simulink model "rectifire_single_inverter_pv1"  (R2022b)
settings: Solver=ode23tb  StartTime=0  StopTime=3  RelTol=1e-4
undefined symbols (not defined in the file): Ion, Lithium, P_100, sigbuilder_block, time_step
libraries: spsSeriesRLCBranchLib x26, spsTriangleGeneratorLib x26, slpidlib x26, spsVoltageMeasurementLib x14, spsCurrentMeasurementLib x11, spsDiodeLib x9, simulink x8, spsIGBTDiodeLib x8, spsMosfetLib x8, powerlib_extras x4, spsGroundLib x2, spsBatteryLib x2
(part 1 of 6)
settings Model: Creator=Administrator  LastModifiedBy=Loki

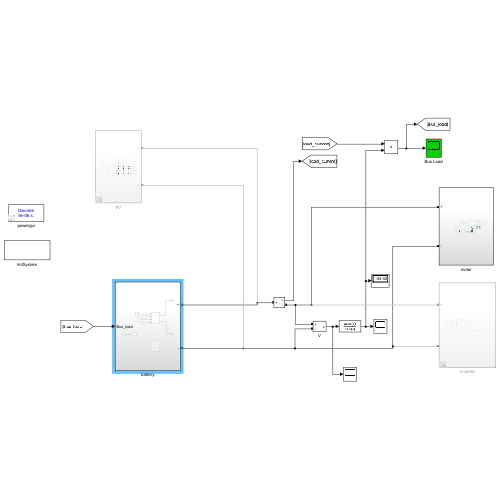
[thumbnail: Simulink's stored preview of the top-level diagram]
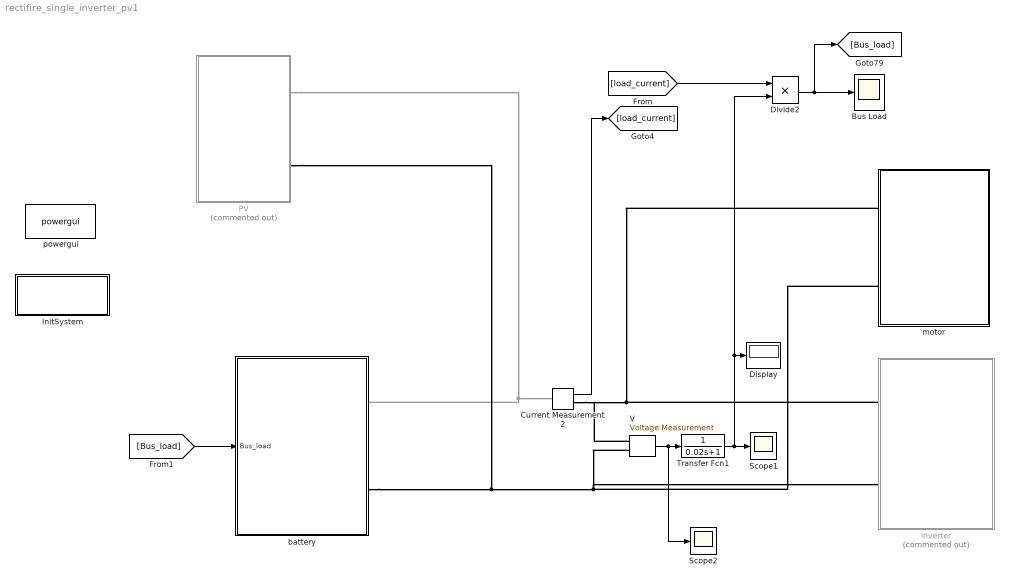
== system rectifire_single_inverter_pv1 ==
  Bus Load : Scope
  Current Measurement2 : spsCurrentMeasurementLib/Current Measurement  PhasorSimulation=off  OutputType=Complex  PSBequivalent=0
  Display : Display
  Divide2 : Product  Inputs=**
  InitSystem : Subsystem
      settings: OpenFcn=Battery_charge_discharge_FSBB_param_init
  PV : Subsystem  Commented=on
  Scope1 : Scope
  Scope2 : Scope
  Transfer Fcn1 : TransferFcn  Denominator=[0.02 1]
  V : spsVoltageMeasurementLib/Voltage Measurement  PhasorSimulation=off  OutputType=Complex  PSBequivalent=0
  battery : Subsystem
  inverter : Subsystem  Commented=on
  motor : Subsystem
  powergui : sps_lib/powergui  Priority=1  SimulationMode=Discrete  SampleTime=5e-6  frequency=60  Iterations=50  frequencyindice=0  Pbase=100e6  ErrMax=1e-4  UnitsV=kV  UnitsW=MW  buscounter=0  FunctionMessages=off  echomessages=off  EnableUseOfTLC=off  CurrentSourceSwitches=off  DisableSnubberDevices=off  DisableRonSwitches=off  DisableVfSwitches=off  DisplayEquations=off  AutomaticDiscreteSolvers=off  SolverType=Tustin/Backward Euler (TBE)  Interpol=off  ExternalGateDelay=off  methode=off  Ts=100  x0status=blocks  SPID=on  SwTol=0  HookPort=off  NonlinearTolerance=1e-4  nMaxIteration=100  ContinueOnMaxIteration=off  RestoreLinks=warning  ResistiveCurrentMeasurement=off  Frange=[0:2:500]  Ylog=off  Xlog=on  ShowGrid=off  save=off  variable=ZData  structure=0  ZoomFFT=off  StartTime=0.0  cycles=1  DisplayStyle=1  fundamental=60  FreqAxis=off  MaxFrequency=1000  frequencyindicesteady=1  RmsSteady=1  display=off
  wires:
  Transfer Fcn1/1 -> Divide2/2, Display/1, Scope1/1
  V/1 -> Scope2/1, Transfer Fcn1/1
  Current Measurement2/1 -> [load_current]
  [load_current] -> Divide2/1
  Divide2/1 -> Bus Load/1, [Bus_load]
  [Bus_load] -> battery/1(Bus_load)
  connections:
  PV/LConn1 -- battery/RConn1 -- Current Measurement2/LConn1
  battery/RConn2 -- motor/LConn2 -- inverter/LConn2 -- V/LConn2 -- PV/LConn2
  motor/LConn1 -- V/LConn1 -- Current Measurement2/RConn1 -- inverter/LConn1

== system rectifire_single_inverter_pv1/InitSystem ==

== system rectifire_single_inverter_pv1/PV ==
  C : spsSeriesRLCBranchLib/Series RLC Branch  LConnTagsString=__new0  RConnTagsString=__new0  BranchType=C  Resistance=0  Inductance=0  SetiL0=off  InitialCurrent=0  Capacitance=300e-6  Setx0=on  InitialVoltage=0  Measurements=None
  C1 : spsSeriesRLCBranchLib/Series RLC Branch  LConnTagsString=__new0  RConnTagsString=__new0  BranchType=C  Resistance=0  Inductance=0  SetiL0=off  InitialCurrent=0  Capacitance=300e-6  Setx0=off  InitialVoltage=0  Measurements=None
  Current Measurement : spsCurrentMeasurementLib/Current Measurement  PhasorSimulation=off  OutputType=Complex  PSBequivalent=0
  G : Subsystem  Tag=STV Subsys  LoadFcn=sigbuilder_block('load');  StartFcn=sigbuilder_block('start');  StopFcn=sigbuilder_block('stop');  ClipboardFcn=sigbuilder_block('clipboard');  mask(Sigbuilder block){tuvar=[0:10]}
      mask help: Sigbuilder GUI
      mask init:
      | if ~strcmp(get_param(bdroot(gcbh),'SimulationStatus'),'stopped') tuvar = sigbuilder_block('maskInit'); end
      settings: CopyFcn=sigbuilder_block('copy');  DeleteFcn=sigbuilder_block('delete');  ModelCloseFcn=sigbuilder_block('modelClose');  PreSaveFcn=sigbuilder_block('preSave');  PauseFcn=sigbuilder_block('pause')  ContinueFcn=sigbuilder_block('continue')  NameChangeFcn=sigbuilder_block('namechange');  OpenFcn=sigbuilder_block('open',[291 78 519 442.2 ]);  CloseFcn=sigbuilder_block('close');
      mask Display: plot(0, 0, 100, 100,[2, 2, 32, 32, 2], [68, 8, 8, 68, 68],[32, 2], [38, 38], [32, 19, 2],[53, 60, 44], [32, 17, 17, 2],[16, 16, 31, 31]);txt = getActiveGroup(gcbh);text(2, 100, txt,'verticalAlignment', 'top');
  Ground : spsGroundLib/Ground  LConnTagsString=a
  IGBT : spsIGBTLib/IGBT  Ron=0.00000001  Lon=0  Vf=1  Tf=1e-6  Tt=2e-6  IC=0  Rs=1e5  Cs=inf  Measurements=off
  L : spsSeriesRLCBranchLib/Series RLC Branch  LConnTagsString=__new0  RConnTagsString=__new0  BranchType=L  Resistance=0  Inductance=200e-6  SetiL0=off  InitialCurrent=1  Capacitance=inf  Setx0=off  InitialVoltage=0  Measurements=None
  "MPPT " : Subsystem
  PV module : Subsystem
  PWM : Subsystem
  R : spsSeriesRLCBranchLib/Series RLC Branch  Commented=on  LConnTagsString=__new0  RConnTagsString=__new0  BranchType=R  Resistance=30  Inductance=100e-6  SetiL0=off  InitialCurrent=0  Capacitance=inf  Setx0=off  InitialVoltage=0  Measurements=None
  Scope : Scope
  T : Subsystem  Tag=STV Subsys  LoadFcn=sigbuilder_block('load');  StartFcn=sigbuilder_block('start');  StopFcn=sigbuilder_block('stop');  ClipboardFcn=sigbuilder_block('clipboard');  mask(Sigbuilder block){tuvar=[0:10]}
      mask help: Sigbuilder GUI
      mask init:
      | if ~strcmp(get_param(bdroot(gcbh),'SimulationStatus'),'stopped') tuvar = sigbuilder_block('maskInit'); end
      settings: CopyFcn=sigbuilder_block('copy');  DeleteFcn=sigbuilder_block('delete');  ModelCloseFcn=sigbuilder_block('modelClose');  PreSaveFcn=sigbuilder_block('preSave');  PauseFcn=sigbuilder_block('pause')  ContinueFcn=sigbuilder_block('continue')  NameChangeFcn=sigbuilder_block('namechange');  OpenFcn=sigbuilder_block('open',[317 199.5 519.5 400 ]);  CloseFcn=sigbuilder_block('close');
      mask Display: plot(0, 0, 100, 100,[2, 2, 32, 32, 2], [68, 8, 8, 68, 68],[32, 2], [38, 38], [32, 19, 2],[53, 60, 44], [32, 17, 17, 2],[16, 16, 31, 31]);txt = getActiveGroup(gcbh);text(2, 100, txt,'verticalAlignment', 'top');
  Terminator{1..4} (4 alike) : Terminator
  VD : spsDiodeLib/Diode  Ron=0.00000001  Lon=0  Vf=0.7  IC=0  UseSnubber=off  Rs=500  Cs=250e-9  Measurements=off
  Voltage Measurement : spsVoltageMeasurementLib/Voltage Measurement  PhasorSimulation=off  OutputType=Complex  PSBequivalent=0
  Voltage Measurement1 : spsVoltageMeasurementLib/Voltage Measurement  PhasorSimulation=off  OutputType=Complex  PSBequivalent=0
  + : PMIOPort  Side=Left
  - : PMIOPort  Port=2  Side=Left
  wires:
  "MPPT "/4(D) -> Terminator1/1, PWM/1(D)  "D"
  Voltage Measurement1/1 -> Scope/1
  "MPPT "/3(I) -> Terminator4/1  "I"
  T/1(Signal 2) -> PV module/1(T)  "T"
  Current Measurement/1 -> "MPPT "/1(i)
  "MPPT "/2(U) -> Terminator3/1  "U"
  "MPPT "/1(P) -> Terminator2/1  "P"
  PWM/1(PWM) -> IGBT/1
  Voltage Measurement/1 -> PV module/3(Load Voltage), "MPPT "/2(u)
  G/1(Signal 1) -> PV module/2(G)  "G"
  connections:
  IGBT/RConn1 -- C/RConn1 -- -/RConn1 -- Voltage Measurement1/LConn2 -- R/RConn1 -- Voltage Measurement/LConn2 -- PV module/LConn1 -- Ground/LConn1 -- C1/RConn1
  R/LConn1 -- Voltage Measurement1/LConn1 -- +/RConn1 -- C/LConn1 -- VD/RConn1
  C1/LConn1 -- L/LConn1 -- Current Measurement/RConn1 -- Voltage Measurement/LConn1
  IGBT/LConn1 -- VD/LConn1 -- L/RConn1
  PV module/RConn1 -- Current Measurement/LConn1

== system rectifire_single_inverter_pv1/battery ==
  Bus_load : Inport
  Battery and DC-DC converter : Subsystem  Commented=on
  Battery and DC-DC converter1 : Subsystem
  Charge0 /Discharge1 : Step  Time=0.3  Before=1  SampleTime=0
  Constant19 : Constant  Value=96
  Constant2 : Constant  Value=30
  + : PMIOPort  Side=Right
  - : PMIOPort  Port=2  Side=Right
  wires:
  Bus_load/1 -> [Bus_load]
  [Bus_load] -> Battery and DC-DC converter1/4(Bus_load)
  Charge0 /Discharge1/1 -> Battery and DC-DC converter1/1(Mode=Charge0/DIscharge1)
  Constant2/1 -> Battery and DC-DC converter1/2(battery_I_charge_ref)
  Constant19/1 -> Battery and DC-DC converter1/3(V_bus_ref)
  connections:
  Battery and DC-DC converter1/RConn1 -- +/RConn1
  Battery and DC-DC converter1/RConn2 -- -/RConn1

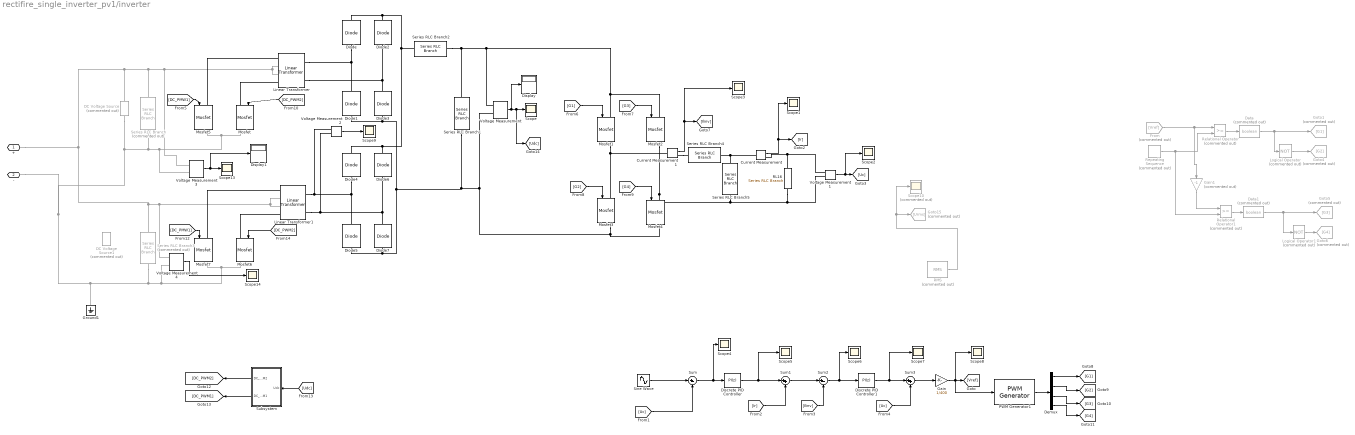
== system rectifire_single_inverter_pv1/inverter ==
  Current Measurement : spsCurrentMeasurementLib/Current Measurement  PhasorSimulation=off  OutputType=Complex  PSBequivalent=0
  Current Measurement1 : spsCurrentMeasurementLib/Current Measurement  PhasorSimulation=off  OutputType=Complex  PSBequivalent=0
  DC Voltage Source : spsDCVoltageSourceLib/DC Voltage Source  Commented=on  Amplitude=96  Measurements=None
  DC Voltage Source1 : spsDCVoltageSourceLib/DC Voltage Source  Commented=on  Amplitude=96  Measurements=None
  Data : DataTypeConversion  Commented=on  OutDataTypeStr=boolean  SaturateOnIntegerOverflow=off  RndMeth=Floor
  Data1 : DataTypeConversion  Commented=on  OutDataTypeStr=boolean  SaturateOnIntegerOverflow=off  RndMeth=Floor
  Demux : Demux
  Diode{,1..7} (8 alike) : spsDiodeLib/Diode  Ron=0.001  Lon=0  Vf=0.8  IC=0  UseSnubber=0  Rs=500  Cs=250e-9  Measurements=off
  Discrete PID Controller : slpidlib/PID Controller  Controller=PI  Form=Parallel  TimeDomain=Discrete-time  UseExternalTs=off  SampleTime=-1  IntegratorMethod=Forward Euler  FilterMethod=Forward Euler  ControllerParametersSource=internal  P=0.03115  I=21  UseKiTs=off  D=0  N=100  UseFilter=on  TunerSelectOption=Transfer Function Based (PID Tuner App)  InitialConditionSource=internal  InitialConditionForIntegrator=0  InitialConditionForFilter=0  DifferentiatorICPrevScaledInput=0  ExternalReset=none  TrackingMode=off  Kt=1  LimitOutput=off  SatLimitsSource=internal  UpperSaturationLimit=inf  LowerSaturationLimit=-inf  LinearizeAsGain=off  AntiWindupMode=none  Kb=1  LimitIntegrator=off  UpperIntegratorSaturationLimit=inf  LowerIntegratorSaturationLimit=-inf  POutMin=[]  POutMax=[]  IOutMin=[]  IOutMax=[]  DOutMin=[]  DOutMax=[]  NOutMin=[]  NOutMax=[]  SumOutMin=[]  SumOutMax=[]  SaturationOutMin=[]  SaturationOutMax=[]  PParamMin=[]  PParamMax=[]  IParamMin=[]  IParamMax=[]  DParamMin=[]  DParamMax=[]  NParamMin=[]  NParamMax=[]  KbParamMin=[]  KbParamMax=[]  KtParamMin=[]  KtParamMax=[]  KbOutMin=[]  KbOutMax=[]  KtOutMin=[]  KtOutMax=[]  IntegratorOutMin=[]  IntegratorOutMax=[]  FilterOutMin=[]  FilterOutMax=[]  SumI1OutMin=[]  SumI1OutMax=[]  SumI2OutMin=[]  SumI2OutMax=[]  SumI3OutMin=[]  SumI3OutMax=[]  SumI4OutMin=[]  SumI4OutMax=[]  SumDOutMin=[]  SumDOutMax=[]  DifferentiatorOutMin=[]  DifferentiatorOutMax=[]  FilterDiffOutCoefMin=[]  FilterDiffOutCoefMax=[]  ReciprocalOutMin=[]  ReciprocalOutMax=[]  SumDenOutMin=[]  SumDenOutMax=[]  SumNumOutMin=[]  SumNumOutMax=[]  DivideOutMin=[]  DivideOutMax=[]  UdiffTsProdOutMin=[]  UdiffTsProdOutMax=[]  NTsProdOutMin=[]  NTsProdOutMax=[]  UintegralTsProdOutMin=[]  UintegralTsProdOutMax=[]  UngainTsProdOutMin=[]  UngainTsProdOutMax=[]  ClampingZeroOutDataTypeStr=Inherit: Inherit via back propagation  ClampingZeroOutMin=[]  ClampingZeroOutMax=[]  FilterDenConstantOutDataTypeStr=Inherit: Inherit via back propagation  FilterDenConstantOutMin=[]  FilterDenConstantOutMax=[]  PCopyOutDataTypeStr=Inherit: Inherit via back propagation  PCopyOutMin=[]  PCopyOutMax=[]  NCopyOutDataTypeStr=Inherit: Inherit via back propagation  NCopyOutMin=[]  NCopyOutMax=[]  IntegratorContinuousStateAttributes=''  IntegratorStateMustResolveToSignalObject=off  IntegratorRTWStateStorageClass=Auto  FilterContinuousStateAttributes=''  FilterStateMustResolveToSignalObject=off  FilterRTWStateStorageClass=Auto  ParallelPVariant=InternalParameters  IdealPVariant=Disabled  IVariant=InternalParameters  DVariant=Disabled  IntegratorVariant=Discrete  SatVariant=Disabled  AWVariant=Passthrough  PCopyVariant=Disabled  TRVariant=Disabled  FdbkBlocksVariant=Forward  IdealPFdbkVariant=Disabled  SatFdbkVariant=Disabled  DerivativeFilterVariant=Disabled  NVariant=Disabled  NCopyVariant=Disabled_SignalSpec  FilterICVariant=Disabled  IntegratorICVariant=InternalICs  ExternalResetVariant=Disabled  TRSumVariant=Passthrough  SumFdbkVariant=Disabled  SumVariant=Sum_PI  TsampFilterVariant=InternalTs  TsampNgainVariant=Passthrough  TsampIntegralVariant=Passthrough  ExternalSaturationOutDataTypeStr=Inherit: Same as second input
      settings: LibrarySourceBlock=simulink/Discrete/Discrete PID Controller
  Discrete PID Controller1 : slpidlib/PID Controller  Controller=PI  Form=Parallel  TimeDomain=Discrete-time  UseExternalTs=off  SampleTime=-1  IntegratorMethod=Forward Euler  FilterMethod=Forward Euler  ControllerParametersSource=internal  P=27.066  I=6.67  UseKiTs=off  D=0  N=100  UseFilter=on  TunerSelectOption=Transfer Function Based (PID Tuner App)  InitialConditionSource=internal  InitialConditionForIntegrator=0  InitialConditionForFilter=0  DifferentiatorICPrevScaledInput=0  ExternalReset=none  TrackingMode=off  Kt=1  LimitOutput=off  SatLimitsSource=internal  UpperSaturationLimit=inf  LowerSaturationLimit=-inf  LinearizeAsGain=off  AntiWindupMode=none  Kb=1  LimitIntegrator=off  UpperIntegratorSaturationLimit=inf  LowerIntegratorSaturationLimit=-inf  POutMin=[]  POutMax=[]  IOutMin=[]  IOutMax=[]  DOutMin=[]  DOutMax=[]  NOutMin=[]  NOutMax=[]  SumOutMin=[]  SumOutMax=[]  SaturationOutMin=[]  SaturationOutMax=[]  PParamMin=[]  PParamMax=[]  IParamMin=[]  IParamMax=[]  DParamMin=[]  DParamMax=[]  NParamMin=[]  NParamMax=[]  KbParamMin=[]  KbParamMax=[]  KtParamMin=[]  KtParamMax=[]  KbOutMin=[]  KbOutMax=[]  KtOutMin=[]  KtOutMax=[]  IntegratorOutMin=[]  IntegratorOutMax=[]  FilterOutMin=[]  FilterOutMax=[]  SumI1OutMin=[]  SumI1OutMax=[]  SumI2OutMin=[]  SumI2OutMax=[]  SumI3OutMin=[]  SumI3OutMax=[]  SumI4OutMin=[]  SumI4OutMax=[]  SumDOutMin=[]  SumDOutMax=[]  DifferentiatorOutMin=[]  DifferentiatorOutMax=[]  FilterDiffOutCoefMin=[]  FilterDiffOutCoefMax=[]  ReciprocalOutMin=[]  ReciprocalOutMax=[]  SumDenOutMin=[]  SumDenOutMax=[]  SumNumOutMin=[]  SumNumOutMax=[]  DivideOutMin=[]  DivideOutMax=[]  UdiffTsProdOutMin=[]  UdiffTsProdOutMax=[]  NTsProdOutMin=[]  NTsProdOutMax=[]  UintegralTsProdOutMin=[]  UintegralTsProdOutMax=[]  UngainTsProdOutMin=[]  UngainTsProdOutMax=[]  ClampingZeroOutDataTypeStr=Inherit: Inherit via back propagation  ClampingZeroOutMin=[]  ClampingZeroOutMax=[]  FilterDenConstantOutDataTypeStr=Inherit: Inherit via back propagation  FilterDenConstantOutMin=[]  FilterDenConstantOutMax=[]  PCopyOutDataTypeStr=Inherit: Inherit via back propagation  PCopyOutMin=[]  PCopyOutMax=[]  NCopyOutDataTypeStr=Inherit: Inherit via back propagation  NCopyOutMin=[]  NCopyOutMax=[]  IntegratorContinuousStateAttributes=''  IntegratorStateMustResolveToSignalObject=off  IntegratorRTWStateStorageClass=Auto  FilterContinuousStateAttributes=''  FilterStateMustResolveToSignalObject=off  FilterRTWStateStorageClass=Auto  ParallelPVariant=InternalParameters  IdealPVariant=Disabled  IVariant=InternalParameters  DVariant=Disabled  IntegratorVariant=Discrete  SatVariant=Disabled  AWVariant=Passthrough  PCopyVariant=Disabled  TRVariant=Disabled  FdbkBlocksVariant=Forward  IdealPFdbkVariant=Disabled  SatFdbkVariant=Disabled  DerivativeFilterVariant=Disabled  NVariant=Disabled  NCopyVariant=Disabled_SignalSpec  FilterICVariant=Disabled  IntegratorICVariant=InternalICs  ExternalResetVariant=Disabled  TRSumVariant=Passthrough  SumFdbkVariant=Disabled  SumVariant=Sum_PI  TsampFilterVariant=InternalTs  TsampNgainVariant=Passthrough  TsampIntegralVariant=Passthrough  ExternalSaturationOutDataTypeStr=Inherit: Same as second input
      settings: LibrarySourceBlock=simulink/Discrete/Discrete PID Controller
  Display : Display
  Display1 : Display
  From : From  Commented=on  GotoTag=Vref
  Gain : Gain  Gain=1/400
  Gain1 : Gain  Commented=on  Gain=-1
  Goto1 : Goto  Commented=on  GotoTag=G1
  Goto15 : Goto  Commented=on  GotoTag=Urms
  Goto4 : Goto  Commented=on  GotoTag=G2
  Goto5 : Goto  Commented=on  GotoTag=G3
  Goto6 : Goto  Commented=on  GotoTag=G4
  Ground1 : spsGroundLib/Ground  LConnTagsString=a
  Linear Transformer : spsLinearTransformerLib/Linear Transformer  UNITS=SI  NominalPower=[ 3000 60 ]  winding1=[96 0 1e-6]  winding2=[96 0 1e-6]  ThreeWindings=on  winding3=[24 0 5e-6]  RmLm=[1.0804e+06 2866]  Measurements=None  DataType=on
  Linear Transformer1 : spsLinearTransformerLib/Linear Transformer  UNITS=SI  NominalPower=[ 3000 60 ]  winding1=[96 0 1e-6]  winding2=[96 0 1e-6]  ThreeWindings=on  winding3=[24 0 5e-6]  RmLm=[1.0804e+06 2866]  Measurements=None  DataType=on
  Logical Operator : Logic  Commented=on  Operator=NOT  AllPortsSameDT=off  OutDataTypeStr=boolean
  Logical Operator1 : Logic  Commented=on  Operator=NOT  AllPortsSameDT=off  OutDataTypeStr=boolean
  Mosfet{,1..7} (8 alike) : spsMosfetLib/Mosfet  Ron=0.1  Lon=0  Rd=0.01  Vfd=0  IC=0  Rs=1e5  Cs=inf  Measurements=on
  PWM Generator1 : powerlib_extras/Control  Blocks/PWM Generator  GeneratorMode="2-arm  bridge (4 pulses)"  Fc=10000  Internal=off  mIndex=0.4  Freq=60  Phase=0
      link override Triangle: rep_seq_y=[0 -1 1 0]
  RL16 : spsSeriesRLCBranchLib/Series RLC Branch  LConnTagsString=__new0  RConnTagsString=__new0  BranchType=R  Resistance=100  Inductance=1e-3  SetiL0=off  InitialCurrent=0  Capacitance=3000e-6  Setx0=off  InitialVoltage=0  Measurements=None
  RMS : spsRMSLib/RMS  Commented=on  TrueRMS=on  Freq=50  RMSInit=0  Ts=0
  Relational Operator : RelationalOperator  Commented=on  OutDataTypeStr=boolean  RndMeth=Simplest  InputSameDT=off
  Relational Operator1 : RelationalOperator  Commented=on  OutDataTypeStr=boolean  RndMeth=Simplest  InputSameDT=off
  Repeating Sequence : simulink/Sources/Repeating Sequence  Commented=on  rep_seq_t=[0 1/20000 1/10000]  rep_seq_y=[-1 1 -1]
  Scope{,1..9,13..14} (12 alike) : Scope
  Scope10 : Scope  Commented=on
  Series RLC Branch : spsSeriesRLCBranchLib/Series RLC Branch  Commented=on  LConnTagsString=__new0  RConnTagsString=__new0  BranchType=C  Resistance=1  Inductance=1e-3  SetiL0=off  InitialCurrent=0  Capacitance=1e-3  Setx0=off  InitialVoltage=0  Measurements=None
  Series RLC Branch1 : spsSeriesRLCBranchLib/Series RLC Branch  LConnTagsString=__new0  RConnTagsString=__new0  BranchType=C  Resistance=1  Inductance=1e-3  SetiL0=off  InitialCurrent=0  Capacitance=500e-6  Setx0=off  InitialVoltage=0  Measurements=None
  Series RLC Branch2 : spsSeriesRLCBranchLib/Series RLC Branch  LConnTagsString=__new0  RConnTagsString=__new0  BranchType=L  Resistance=1  Inductance=2e-3  SetiL0=off  InitialCurrent=0  Capacitance=1e-6  Setx0=off  InitialVoltage=0  Measurements=None
  Series RLC Branch3 : spsSeriesRLCBranchLib/Series RLC Branch  Commented=on  LConnTagsString=__new0  RConnTagsString=__new0  BranchType=C  Resistance=1  Inductance=1e-3  SetiL0=off  InitialCurrent=0  Capacitance=1e-3  Setx0=off  InitialVoltage=0  Measurements=None
  Series RLC Branch4 : spsSeriesRLCBranchLib/Series RLC Branch  LConnTagsString=__new0  RConnTagsString=__new0  BranchType=L  Resistance=0  Inductance=4.06e-3  SetiL0=off  InitialCurrent=0  Capacitance=1e-6  Setx0=off  InitialVoltage=0  Measurements=None
  Series RLC Branch5 : spsSeriesRLCBranchLib/Series RLC Branch  LConnTagsString=__new0  RConnTagsString=__new0  BranchType=C  Resistance=1  Inductance=1e-3  SetiL0=off  InitialCurrent=0  Capacitance=6.23e-6  Setx0=off  InitialVoltage=0  Measurements=None
  Sine Wave : Sin  Amplitude=311  Frequency=100*pi  SampleTime=0
  Subsystem : Subsystem
  Sum : Sum  Inputs=|+-
  Sum1 : Sum  Inputs=|++
  Sum2 : Sum  Inputs=|+-
  Sum3 : Sum  Inputs=|++
  Voltage Measurement{,1..4} (5 alike) : spsVoltageMeasurementLib/Voltage Measurement  PhasorSimulation=off  OutputType=Complex  PSBequivalent=0
  + : PMIOPort  Side=Left
  - : PMIOPort  Port=2  Side=Left
  wires:
  Current Measurement1/1 -> Scope3/1, [Ilinv]
  Logical Operator1/1 -> Goto6/1
  [G4] -> Mosfet4/1
  Repeating Sequence/1 -> Relational Operator1/2, Relational Operator/2
  Gain/1 -> PWM Generator1/1, Scope8/1, [Vref]
  [Ilinv] -> Sum2/2
  Voltage Measurement1/1 -> Scope2/1, [Uc]
  Sum1/1 -> Sum2/1
  [G3] -> Mosfet2/1
  Discrete PID Controller1/1 -> Scope7/1, Sum3/1
  RMS/1 -> Scope10/1, Goto15/1
  Voltage Measurement4/1 -> Scope14/1
  [DC_PWM2] -> Mosfet6/1
  Gain1/1 -> Relational Operator1/1
  Demux/3 -> [G3]
  [DC_PMW1] -> Mosfet7/1
  [G2] -> Mosfet3/1
  Sum/1 -> Scope4/1, Discrete PID Controller/1
  Relational Operator/1 -> Data/1
  Sine Wave/1 -> Sum/1
  Relational Operator1/1 -> Data1/1
  Data/1 -> Logical Operator/1, Goto1/1
  Sum3/1 -> Gain/1
  From/1 -> Gain1/1, Relational Operator/1
  Voltage Measurement3/1 -> Display1/1, Scope13/1
  Voltage Measurement/1 -> Display/1, [Udc], Scope/1
  [Uc] -> Sum3/2
  [Ir] -> Sum1/2
  [DC_PMW1] -> Mosfet5/1
  Current Measurement/1 -> Scope1/1, [Ir]
  Logical Operator/1 -> Goto4/1
  Sum2/1 -> Scope6/1, Discrete PID Controller1/1
  PWM Generator1/1 -> Demux/1
  [G1] -> Mosfet1/1
  Discrete PID Controller/1 -> Scope5/1, Sum1/1
  Demux/1 -> [G1]
  Demux/4 -> [G4]
  [DC_PWM2] -> Mosfet/1
  Voltage Measurement2/1 -> Scope9/1
  Data1/1 -> Logical Operator1/1, Goto5/1
  Demux/2 -> [G2]
  [Uc] -> Sum/2
  [Udc] -> Subsystem/1(Udc)
  Subsystem/1(DC_PWM2) -> [DC_PWM2]
  Subsystem/2(DC_PWM1) -> [DC_PWM1]
  connections:
  RL16/RConn1 -- Voltage Measurement1/LConn2 -- Series RLC Branch5/RConn1 -- Mosfet2/RConn1 -- Mosfet4/LConn1
  Linear Transformer/LConn1 -- Diode1/RConn1 -- Diode/LConn1
  Diode4/LConn1 -- Diode5/RConn1 -- Voltage Measurement2/LConn1 -- Linear Transformer1/LConn1
  Current Measurement/LConn1 -- Series RLC Branch5/LConn1 -- Series RLC Branch4/LConn1
  Voltage Measurement/LConn2 -- Mosfet3/RConn1 -- Mosfet4/RConn1 -- Series RLC Branch1/RConn1 -- Diode5/LConn1 -- Diode7/LConn1 -- Diode1/LConn1 -- Diode3/LConn1
  Mosfet1/RConn1 -- Current Measurement1/LConn1 -- Mosfet3/LConn1
  Diode7/RConn1 -- Diode6/LConn1 -- Voltage Measurement2/LConn2 -- Linear Transformer1/LConn2
  Voltage Measurement/LConn1 -- Series RLC Branch2/LConn1 -- Series RLC Branch1/LConn1 -- Mosfet1/LConn1 -- Mosfet2/LConn1
  Series RLC Branch/LConn1 -- Voltage Measurement3/LConn1 -- Linear Transformer/RConn3 -- Linear Transformer/RConn2 -- DC Voltage Source/RConn1 -- Series RLC Branch3/LConn1 -- Voltage Measurement4/LConn1 -- Linear Transformer1/RConn2 -- Linear Transformer1/RConn3 -- +/RConn1
  Diode6/RConn1 -- Series RLC Branch2/RConn1 -- Diode/RConn1 -- Diode2/RConn1 -- Diode4/RConn1
  Linear Transformer/LConn2 -- Diode2/LConn1 -- Diode3/RConn1
  RL16/LConn1 -- Voltage Measurement1/LConn1 -- Current Measurement/RConn1
  DC Voltage Source/LConn1 -- -/RConn1 -- Ground1/LConn1 -- Series RLC Branch3/RConn1 -- Voltage Measurement4/LConn2 -- Mosfet7/RConn1 -- Mosfet6/RConn1 -- Mosfet5/RConn1 -- Mosfet/RConn1 -- Voltage Measurement3/LConn2 -- Series RLC Branch/RConn1
  Current Measurement1/RConn1 -- Series RLC Branch4/RConn1
  Linear Transformer1/RConn1 -- Mosfet7/LConn1
  Mosfet5/LConn1 -- Linear Transformer/RConn1
  Mosfet/LConn1 -- Linear Transformer/RConn4
  Linear Transformer1/RConn4 -- Mosfet6/LConn1

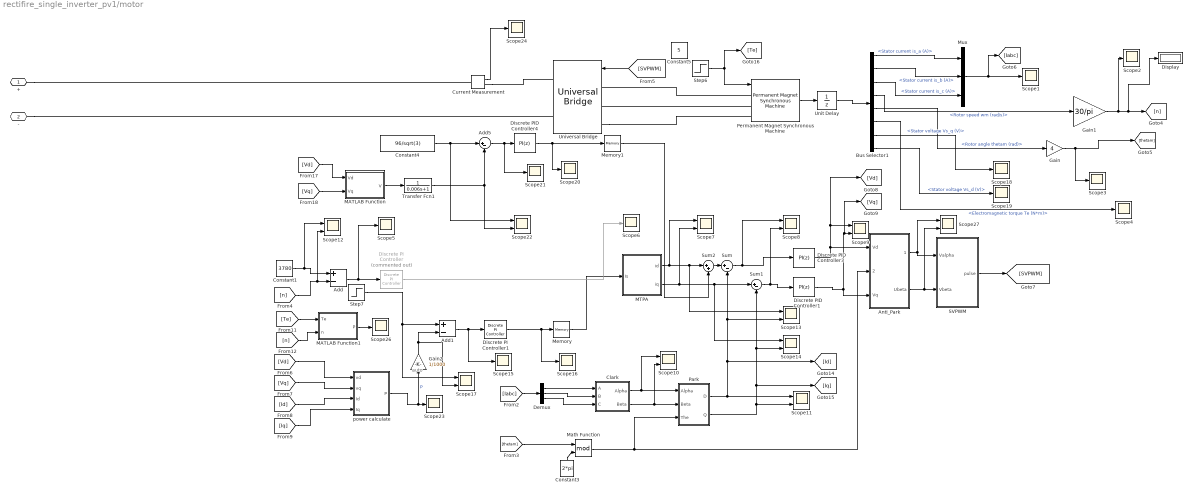
== system rectifire_single_inverter_pv1/motor ==
  note: auto
  Add : Sum  Inputs=+-
  Add1 : Sum  Inputs=+-
  Add5 : Sum  Inputs=|+-
  Anti_Park : Subsystem
  Bus Selector1 : BusSelector  OutputSignals=Stator current is_a (A),Stator current is_b (A),Stator current is_c (A),Rotor speed wm (rad/s),Rotor angle thetam (rad),Electromagnetic torque Te (N*m),Stator voltage Vs_q (V),Stator voltage Vs_d (V)
  Clark : Subsystem
  Constant1 : Constant  Value=3780
  Constant3 : Constant  Value=2*pi  SampleTime=5e-6
  Constant4 : Constant  Value=96/sqrt(3)
  Constant5 : Constant  Value=5
  Current Measurement : spsCurrentMeasurementLib/Current Measurement  PhasorSimulation=off  OutputType=Complex  PSBequivalent=0
  Demux : Demux  Outputs=3
  Discrete PI Controller : powerlib_extras/Discrete  Control Blocks/Discrete PI Controller  Commented=on  Kp=1.7  Ki=0.2  Par_Limits=[100 -100]  Init=0  Ts=5e-6
  Discrete PI Controller1 : powerlib_extras/Discrete  Control Blocks/Discrete PI Controller  Kp=20  Ki=500  Par_Limits=[inf -inf]  Init=0  Ts=5e-6
  Discrete PID Controller1 : slpidlib/PID Controller  Controller=PI  Form=Parallel  TimeDomain=Discrete-time  UseExternalTs=off  SampleTime=5e-6  IntegratorMethod=Forward Euler  FilterMethod=Forward Euler  ControllerParametersSource=internal  P=1.2  I=0.1  UseKiTs=off  D=0  N=100  UseFilter=on  TunerSelectOption=Transfer Function Based (PID Tuner App)  InitialConditionSource=internal  InitialConditionForIntegrator=0  InitialConditionForFilter=0  DifferentiatorICPrevScaledInput=0  ExternalReset=none  TrackingMode=off  Kt=1  LimitOutput=on  SatLimitsSource=internal  UpperSaturationLimit=50  LowerSaturationLimit=-50  LinearizeAsGain=off  AntiWindupMode=none  Kb=1  LimitIntegrator=off  UpperIntegratorSaturationLimit=inf  LowerIntegratorSaturationLimit=-inf  POutMin=[]  POutMax=[]  IOutMin=[]  IOutMax=[]  DOutMin=[]  DOutMax=[]  NOutMin=[]  NOutMax=[]  SumOutMin=[]  SumOutMax=[]  SaturationOutMin=[]  SaturationOutMax=[]  PParamMin=[]  PParamMax=[]  IParamMin=[]  IParamMax=[]  DParamMin=[]  DParamMax=[]  NParamMin=[]  NParamMax=[]  KbParamMin=[]  KbParamMax=[]  KtParamMin=[]  KtParamMax=[]  KbOutMin=[]  KbOutMax=[]  KtOutMin=[]  KtOutMax=[]  IntegratorOutMin=[]  IntegratorOutMax=[]  FilterOutMin=[]  FilterOutMax=[]  SumI1OutMin=[]  SumI1OutMax=[]  SumI2OutMin=[]  SumI2OutMax=[]  SumI3OutMin=[]  SumI3OutMax=[]  SumI4OutMin=[]  SumI4OutMax=[]  SumDOutMin=[]  SumDOutMax=[]  DifferentiatorOutMin=[]  DifferentiatorOutMax=[]  FilterDiffOutCoefMin=[]  FilterDiffOutCoefMax=[]  ReciprocalOutMin=[]  ReciprocalOutMax=[]  SumDenOutMin=[]  SumDenOutMax=[]  SumNumOutMin=[]  SumNumOutMax=[]  DivideOutMin=[]  DivideOutMax=[]  UdiffTsProdOutMin=[]  UdiffTsProdOutMax=[]  NTsProdOutMin=[]  NTsProdOutMax=[]  UintegralTsProdOutMin=[]  UintegralTsProdOutMax=[]  UngainTsProdOutMin=[]  UngainTsProdOutMax=[]  ClampingZeroOutDataTypeStr=Inherit: Inherit via back propagation  ClampingZeroOutMin=[]  ClampingZeroOutMax=[]  FilterDenConstantOutDataTypeStr=Inherit: Inherit via back propagation  FilterDenConstantOutMin=[]  FilterDenConstantOutMax=[]  PCopyOutDataTypeStr=Inherit: Inherit via back propagation  PCopyOutMin=[]  PCopyOutMax=[]  NCopyOutDataTypeStr=Inherit: Inherit via back propagation  NCopyOutMin=[]  NCopyOutMax=[]  IntegratorContinuousStateAttributes=''  IntegratorStateMustResolveToSignalObject=off  IntegratorRTWStateStorageClass=Auto  FilterContinuousStateAttributes=''  FilterStateMustResolveToSignalObject=off  FilterRTWStateStorageClass=Auto  ParallelPVariant=InternalParameters  IdealPVariant=Disabled  IVariant=InternalParameters  DVariant=Disabled  IntegratorVariant=Discrete  SatVariant=Enabled  AWVariant=Passthrough  PCopyVariant=Disabled  TRVariant=Disabled  FdbkBlocksVariant=Forward  IdealPFdbkVariant=Disabled  SatFdbkVariant=Disabled  DerivativeFilterVariant=Disabled  NVariant=Disabled  NCopyVariant=Disabled_SignalSpec  FilterICVariant=Disabled  IntegratorICVariant=InternalICs  ExternalResetVariant=Disabled  TRSumVariant=Passthrough  SumFdbkVariant=Disabled  SumVariant=Sum_PI  TsampFilterVariant=InternalTs  TsampNgainVariant=Passthrough  TsampIntegralVariant=Passthrough  ExternalSaturationOutDataTypeStr=Inherit: Same as second input
  Discrete PID Controller3 : slpidlib/PID Controller  Controller=PI  Form=Parallel  TimeDomain=Discrete-time  UseExternalTs=off  SampleTime=5e-6  IntegratorMethod=Forward Euler  FilterMethod=Forward Euler  ControllerParametersSource=internal  P=1.2  I=0.1  UseKiTs=off  D=0  N=100  UseFilter=on  TunerSelectOption=Transfer Function Based (PID Tuner App)  InitialConditionSource=internal  InitialConditionForIntegrator=0  InitialConditionForFilter=0  DifferentiatorICPrevScaledInput=0  ExternalReset=none  TrackingMode=off  Kt=1  LimitOutput=on  SatLimitsSource=internal  UpperSaturationLimit=50  LowerSaturationLimit=-50  LinearizeAsGain=off  AntiWindupMode=none  Kb=1  LimitIntegrator=off  UpperIntegratorSaturationLimit=inf  LowerIntegratorSaturationLimit=-inf  POutMin=[]  POutMax=[]  IOutMin=[]  IOutMax=[]  DOutMin=[]  DOutMax=[]  NOutMin=[]  NOutMax=[]  SumOutMin=[]  SumOutMax=[]  SaturationOutMin=[]  SaturationOutMax=[]  PParamMin=[]  PParamMax=[]  IParamMin=[]  IParamMax=[]  DParamMin=[]  DParamMax=[]  NParamMin=[]  NParamMax=[]  KbParamMin=[]  KbParamMax=[]  KtParamMin=[]  KtParamMax=[]  KbOutMin=[]  KbOutMax=[]  KtOutMin=[]  KtOutMax=[]  IntegratorOutMin=[]  IntegratorOutMax=[]  FilterOutMin=[]  FilterOutMax=[]  SumI1OutMin=[]  SumI1OutMax=[]  SumI2OutMin=[]  SumI2OutMax=[]  SumI3OutMin=[]  SumI3OutMax=[]  SumI4OutMin=[]  SumI4OutMax=[]  SumDOutMin=[]  SumDOutMax=[]  DifferentiatorOutMin=[]  DifferentiatorOutMax=[]  FilterDiffOutCoefMin=[]  FilterDiffOutCoefMax=[]  ReciprocalOutMin=[]  ReciprocalOutMax=[]  SumDenOutMin=[]  SumDenOutMax=[]  SumNumOutMin=[]  SumNumOutMax=[]  DivideOutMin=[]  DivideOutMax=[]  UdiffTsProdOutMin=[]  UdiffTsProdOutMax=[]  NTsProdOutMin=[]  NTsProdOutMax=[]  UintegralTsProdOutMin=[]  UintegralTsProdOutMax=[]  UngainTsProdOutMin=[]  UngainTsProdOutMax=[]  ClampingZeroOutDataTypeStr=Inherit: Inherit via back propagation  ClampingZeroOutMin=[]  ClampingZeroOutMax=[]  FilterDenConstantOutDataTypeStr=Inherit: Inherit via back propagation  FilterDenConstantOutMin=[]  FilterDenConstantOutMax=[]  PCopyOutDataTypeStr=Inherit: Inherit via back propagation  PCopyOutMin=[]  PCopyOutMax=[]  NCopyOutDataTypeStr=Inherit: Inherit via back propagation  NCopyOutMin=[]  NCopyOutMax=[]  IntegratorContinuousStateAttributes=''  IntegratorStateMustResolveToSignalObject=off  IntegratorRTWStateStorageClass=Auto  FilterContinuousStateAttributes=''  FilterStateMustResolveToSignalObject=off  FilterRTWStateStorageClass=Auto  ParallelPVariant=InternalParameters  IdealPVariant=Disabled  IVariant=InternalParameters  DVariant=Disabled  IntegratorVariant=Discrete  SatVariant=Enabled  AWVariant=Passthrough  PCopyVariant=Disabled  TRVariant=Disabled  FdbkBlocksVariant=Forward  IdealPFdbkVariant=Disabled  SatFdbkVariant=Disabled  DerivativeFilterVariant=Disabled  NVariant=Disabled  NCopyVariant=Disabled_SignalSpec  FilterICVariant=Disabled  IntegratorICVariant=InternalICs  ExternalResetVariant=Disabled  TRSumVariant=Passthrough  SumFdbkVariant=Disabled  SumVariant=Sum_PI  TsampFilterVariant=InternalTs  TsampNgainVariant=Passthrough  TsampIntegralVariant=Passthrough  ExternalSaturationOutDataTypeStr=Inherit: Same as second input
  Discrete PID Controller4 : slpidlib/PID Controller  Controller=PI  Form=Parallel  TimeDomain=Discrete-time  UseExternalTs=off  SampleTime=5e-6  IntegratorMethod=Forward Euler  FilterMethod=Forward Euler  ControllerParametersSource=internal  P=0.02  I=0.000008  UseKiTs=off  D=0  N=100  UseFilter=on  TunerSelectOption=Transfer Function Based (PID Tuner App)  InitialConditionSource=internal  InitialConditionForIntegrator=0  InitialConditionForFilter=0  DifferentiatorICPrevScaledInput=0  ExternalReset=none  TrackingMode=off  Kt=1  LimitOutput=off  SatLimitsSource=internal  UpperSaturationLimit=inf  LowerSaturationLimit=-inf  LinearizeAsGain=off  AntiWindupMode=none  Kb=1  LimitIntegrator=off  UpperIntegratorSaturationLimit=inf  LowerIntegratorSaturationLimit=-inf  POutMin=[]  POutMax=[]  IOutMin=[]  IOutMax=[]  DOutMin=[]  DOutMax=[]  NOutMin=[]  NOutMax=[]  SumOutMin=[]  SumOutMax=[]  SaturationOutMin=[]  SaturationOutMax=[]  PParamMin=[]  PParamMax=[]  IParamMin=[]  IParamMax=[]  DParamMin=[]  DParamMax=[]  NParamMin=[]  NParamMax=[]  KbParamMin=[]  KbParamMax=[]  KtParamMin=[]  KtParamMax=[]  KbOutMin=[]  KbOutMax=[]  KtOutMin=[]  KtOutMax=[]  IntegratorOutMin=[]  IntegratorOutMax=[]  FilterOutMin=[]  FilterOutMax=[]  SumI1OutMin=[]  SumI1OutMax=[]  SumI2OutMin=[]  SumI2OutMax=[]  SumI3OutMin=[]  SumI3OutMax=[]  SumI4OutMin=[]  SumI4OutMax=[]  SumDOutMin=[]  SumDOutMax=[]  DifferentiatorOutMin=[]  DifferentiatorOutMax=[]  FilterDiffOutCoefMin=[]  FilterDiffOutCoefMax=[]  ReciprocalOutMin=[]  ReciprocalOutMax=[]  SumDenOutMin=[]  SumDenOutMax=[]  SumNumOutMin=[]  SumNumOutMax=[]  DivideOutMin=[]  DivideOutMax=[]  UdiffTsProdOutMin=[]  UdiffTsProdOutMax=[]  NTsProdOutMin=[]  NTsProdOutMax=[]  UintegralTsProdOutMin=[]  UintegralTsProdOutMax=[]  UngainTsProdOutMin=[]  UngainTsProdOutMax=[]  ClampingZeroOutDataTypeStr=Inherit: Inherit via back propagation  ClampingZeroOutMin=[]  ClampingZeroOutMax=[]  FilterDenConstantOutDataTypeStr=Inherit: Inherit via back propagation  FilterDenConstantOutMin=[]  FilterDenConstantOutMax=[]  PCopyOutDataTypeStr=Inherit: Inherit via back propagation  PCopyOutMin=[]  PCopyOutMax=[]  NCopyOutDataTypeStr=Inherit: Inherit via back propagation  NCopyOutMin=[]  NCopyOutMax=[]  IntegratorContinuousStateAttributes=''  IntegratorStateMustResolveToSignalObject=off  IntegratorRTWStateStorageClass=Auto  FilterContinuousStateAttributes=''  FilterStateMustResolveToSignalObject=off  FilterRTWStateStorageClass=Auto  ParallelPVariant=InternalParameters  IdealPVariant=Disabled  IVariant=InternalParameters  DVariant=Disabled  IntegratorVariant=Discrete  SatVariant=Disabled  AWVariant=Passthrough  PCopyVariant=Disabled  TRVariant=Disabled  FdbkBlocksVariant=Forward  IdealPFdbkVariant=Disabled  SatFdbkVariant=Disabled  DerivativeFilterVariant=Disabled  NVariant=Disabled  NCopyVariant=Disabled_SignalSpec  FilterICVariant=Disabled  IntegratorICVariant=InternalICs  ExternalResetVariant=Disabled  TRSumVariant=Passthrough  SumFdbkVariant=Disabled  SumVariant=Sum_PI  TsampFilterVariant=InternalTs  TsampNgainVariant=Passthrough  TsampIntegralVariant=Passthrough  ExternalSaturationOutDataTypeStr=Inherit: Same as second input
      settings: LibrarySourceBlock=simulink/Discrete/Discrete PID Controller
  Display : Display
  Gain : Gain  Gain=4
  Gain1 : Gain  Gain=30/pi
  Gain2 : Gain  Gain=1/1000
  MATLAB Function : MATLAB Function  TreatAsAtomicUnit=on
  MATLAB Function1 : MATLAB Function  TreatAsAtomicUnit=on
  MTPA : MATLAB Function  TreatAsAtomicUnit=on
  Math Function : Math  Operator=mod  SignedPower=on
  Memory : Memory
  Memory1 : Memory
  Mux : Mux  Inputs=3
  Park : Subsystem
  Permanent Magnet Synchronous Machine : spsPermanentMagnetSynchronousMachineLib/Permanent Magnet Synchronous Machine  NbPhases=3  FluxDistribution=Sinusoidal  RotorType=Salient-pole  MechanicalLoad=Torque Tm  PresetModel=No  ShowDetailedParameters=on  MeasurementBus=off  Resistance=0.00513  Inductance=8.5e-3  dqInductances=[3.23e-5,5.7e-5]  La=0.000395  MachineConstant=Flux linkage established by magnets (V.s)  Flux=0.00569  VoltageCst=4.1282  TorqueCst=0.03414  Flat=120  Mechanical=[0.0024375 0.00005 4 0]  PolePairs=4  InitialConditions=[0,0, 0,0]  InitialConditions5ph=[0 0 0 0 0 0]  RefAngle=Aligned with phase A axis (original Park)  IterativeDiscreteModel=Trapezoidal non iterative  TsBlock=-1  TsPowergui=0
  SVPWM : Subsystem
  Scope{1..6,15..16,18..21,23..24,26} (15 alike) : Scope
  Scope{7..14,17,22,27} (11 alike) : Scope  NumInputPorts=2
  Step6 : Step  Before=5  After=5  SampleTime=0
  Step7 : Step  Time=0.05  Before=1.6  After=1.6  SampleTime=0
  Sum : Sum  Inputs=|+-
  Sum1 : Sum  Inputs=|+-
  Sum2 : Sum  Inputs=|++
  Transfer Fcn1 : TransferFcn  Denominator=[0.006 1]
  Unit Delay : UnitDelay  SampleTime=-1  HasFrameUpgradeWarning=on
  Universal Bridge : spsUniversalBridgeLib/Universal Bridge  Arms=3  SnubberResistance=1e5  SnubberCapacitance=inf  Device=IGBT / Diodes  Ron=1e-3  Lon=0  ForwardVoltages="[  0  0  ]"  ForwardVoltage=0  GTOparameters=[ 10e-6 , 20e-6 ]  IGBTparameters=[ 1e-6 , 2e-6 ]  Measurements=All voltages and currents  Measurements_2=None  converterType=Rectifier
  power calculate : Subsystem
  + : PMIOPort  Side=Left
  - : PMIOPort  Port=2  Side=Left
  wires:
  MTPA/1(id) -> Scope7/1, Sum2/1, Scope13/1
  Discrete PID Controller3/1 -> [Vd], Scope9/1, Anti_Park/1(Vd)
  Anti_Park/2(Ubeta) -> Scope27/2, SVPWM/2(Vbeta)
  Park/2(Q) -> Scope11/2, [Iq], Scope14/2, Sum1/2
  Sum/1 -> Discrete PID Controller3/1, Scope8/1
  [Te] -> MATLAB Function1/1(Te)
  Anti_Park/1(Ualpha) -> SVPWM/1(Valpha), Scope27/1
  Discrete PI Controller1/1 -> Memory/1, Scope16/1
  [n] -> Scope12/2, Add/2
  Gain/1 -> Scope3/1, [thetam]
  Demux/2 -> Clark/2(B)
  Add/1 -> Discrete PI Controller/1, Scope5/1
  Mux/1 -> [Iabc], Scope1/1
  Memory1/1 -> Sum2/2
  Bus Selector1/1 -> Mux/1  "<Stator current is_a (A)>"
  Bus Selector1/5 -> Gain/1  "<Rotor angle thetam (rad)>"
  Unit Delay/1 -> Bus Selector1/1
  Constant1/1 -> Scope12/1, Add/1
  Bus Selector1/6 -> Scope4/1  "<Electromagnetic torque Te (N*m)>"
  MTPA/2(iq) -> Scope7/2, Scope14/1, Sum1/1
  Discrete PID Controller1/1 -> [Vq], Scope9/2, Anti_Park/3(Vq)
  [n] -> MATLAB Function1/2(n)
  Demux/3 -> Clark/3(C)
  Sum1/1 -> Discrete PID Controller1/1, Scope8/2
  Bus Selector1/3 -> Mux/3  "<Stator current is_c (A)>"
  Memory/1 -> MTPA/1(Is)
  Add5/1 -> Scope21/1, Discrete PID Controller4/1
  [Vq] -> power calculate/2(vq)
  Constant3/1 -> Math Function/2
  Park/1(D) -> Scope11/1, [Id], Scope13/2, Sum/2
  [Vq] -> MATLAB Function/2(Vq)
  power calculate/1(P) -> Gain2/1, Scope23/1  "P"
  Discrete PID Controller4/1 -> Scope20/1, Memory1/1
  Add1/1 -> Scope15/1, Discrete PI Controller1/1
  [Iabc] -> Demux/1
  [Vd] -> MATLAB Function/1(Vd)
  Math Function/1 -> Anti_Park/2(thetam), Park/3(The)
  SVPWM/1(pulse) -> [SVPWM]
  Clark/2(Beta) -> Scope10/2, Park/2(Beta)
  Bus Selector1/8 -> Scope19/1  "<Stator voltage Vs_d (V)>"
  Gain2/1 -> Add1/2, Scope17/2
  Demux/1 -> Clark/1(A)
  Bus Selector1/4 -> Gain1/1  "<Rotor speed wm (rad/s)>"
  Constant4/1 -> Scope22/1, Add5/1
  Step7/1 -> Scope17/1, Add1/1
  [SVPWM] -> Universal Bridge/1
  [Iq] -> power calculate/4(Iq)
  [Id] -> power calculate/3(Id)
  Bus Selector1/2 -> Mux/2  "<Stator current is_b (A)>"
  Discrete PI Controller/1 -> Scope6/1
  Sum2/1 -> Sum/1
  Transfer Fcn1/1 -> Add5/2, Scope22/2
  [thetam] -> Math Function/1
  Current Measurement/1 -> Scope24/1
  Clark/1(Alpha) -> Scope10/1, Park/1(Alpha)
  MATLAB Function/1(V) -> Transfer Fcn1/1
  MATLAB Function1/1(P) -> Scope26/1
  Bus Selector1/7 -> Scope18/1  "<Stator voltage Vs_q (V)>"
  [Vd] -> power calculate/1(vd)
  Gain1/1 -> Scope2/1, Display/1, [n]
  Permanent Magnet Synchronous Machine/1 -> Unit Delay/1
  Step6/1 -> [Te], Permanent Magnet Synchronous Machine/1
  connections:
  Universal Bridge/LConn3 -- Permanent Magnet Synchronous Machine/LConn3
  Permanent Magnet Synchronous Machine/LConn2 -- Universal Bridge/LConn2
  Permanent Magnet Synchronous Machine/LConn1 -- Universal Bridge/LConn1
  Current Measurement/RConn1 -- Universal Bridge/RConn1
  +/RConn1 -- Current Measurement/LConn1
  -/RConn1 -- Universal Bridge/RConn2

== system rectifire_single_inverter_pv1/PV/G ==
  Demux : Demux  Tag=STV Demux  Outputs=1
      settings: DisplayOption=none
  FromWs : FromWorkspace  Tag=STV FromWs  VariableName=tuvar  ZeroCross=off
      SigBuilderData=|
      | dataSet.timeRange = [0 2]
      | dataSet.name = 'Group 1'
      | sbobj.Groups.Name = 'Group 1'
      | sbobj.Groups.Signals.Name = 'Signal 1'
      | sbobj.Groups.Signals.XData = [0 0.0795 0.16 2]
      | sbobj.Groups.Signals.YData = [1000 1149.5 1001 1001]
      | sbobj.Groups.TimeRange = [0 2]
  Signal 1 : Outport  Tag=STV Outport
  wires:
  FromWs/1 -> Demux/1
  Demux/1 -> Signal 1/1

== system rectifire_single_inverter_pv1/PV/MPPT  ==
  i : Inport
  u : Inport  Port=2
  Add : Sum
  Constant2 : Constant  Value=-0.01
  Memory : Memory  InheritSampleTime=on
  Memory1 : Memory  InheritSampleTime=on
  Memory2 : Memory  InitialCondition=1  InheritSampleTime=on
  Product{,1..3} (4 alike) : Product  RndMeth=Zero
  Sign : Signum
  Sign1 : Signum
  Sign2 : Signum
  Subtract : Sum  Inputs=+-
  Subtract1 : Sum  Inputs=+-
  Zero-Order Hold : ZeroOrderHold  SampleTime=0.0005
  Zero-Order Hold1 : ZeroOrderHold  SampleTime=0.0005
  Zero-Order Hold3 : ZeroOrderHold  SampleTime=0.0005
  P : Outport
  U : Outport  Port=2
  I : Outport  Port=3
  D : Outport  Port=4
  wires:
  u/1 -> Zero-Order Hold/1, Product3/2, U/1
  i/1 -> Zero-Order Hold1/1, Product3/1, I/1
  Zero-Order Hold/1 -> Product/1, Subtract/1, Memory/1
  Memory/1 -> Subtract/2
  Zero-Order Hold1/1 -> Product/2
  Product/1 -> Subtract1/1, Memory1/1
  Memory1/1 -> Subtract1/2
  Subtract/1 -> Sign/1
  Subtract1/1 -> Sign1/1
  Sign/1 -> Product1/1
  Sign1/1 -> Product1/2
  Product1/1 -> Sign2/1
  Sign2/1 -> Product2/1
  Add/1 -> Memory2/1, D/1
  Memory2/1 -> Add/2
  Constant2/1 -> Product2/2
  Product3/1 -> P/1
  Product2/1 -> Zero-Order Hold3/1
  Zero-Order Hold3/1 -> Add/1

== system rectifire_single_inverter_pv1/PV/PV module ==
  T : Inport
  G : Inport  Port=2
  Load Voltage : Inport  Port=3
  Controlled Current Source : spsControlledCurrentSourceLib/Controlled Current Source  Initialize=on  Source_Type=AC  Amplitude=0  Phase=0  Frequency=0  Measurements=None
  PV module1 : Subsystem  mask{ki=0.0032, q=1.6e-19, K=1.38e-23, n=1.3, Eg0=1.1, Rs=0.221, Rsh=415.405, Tn=298, Voc=32.9, Isc=8.21, Ns=54}
      mask DialogControl DescGroupVar Prompt: PV Module
      mask DialogControl DescTextVar Prompt: 更改下列参数，以达到仿真效果。
      mask DialogControl ParameterGroupVar Prompt: 参数
  + : PMIOPort  Side=Right
  - : PMIOPort  Port=2  Side=Left
  wires:
  PV module1/1(I) -> Controlled Current Source/1
  Load Voltage/1 -> PV module1/3(Load Voltage)
  T/1 -> PV module1/1(T)
  G/1 -> PV module1/2(G)
  connections:
  -/RConn1 -- Controlled Current Source/LConn1
  Controlled Current Source/RConn1 -- +/RConn1

== system rectifire_single_inverter_pv1/PV/PWM ==
  D : Inport
  Constant : Constant  Commented=on
  Constant1 : Constant  Commented=on  Value=0
  PWM Generator (DC-DC) : spsPWMGeneratorDCDCLib/PWM Generator (DC-DC)  Fsw=5000  Ts=0
  Repeating Sequence : simulink/Sources/Repeating Sequence  Commented=on  rep_seq_t=[0 0.0001]  rep_seq_y=[0 1]
  Saturation : Saturate  Commented=on  UpperLimit=1  LowerLimit=0
  Subtract2 : Sum  Commented=on  Inputs=+-
  Switch : Switch  Commented=on  SaturateOnIntegerOverflow=off  InputSameDT=off
  Zero-Order Hold2 : ZeroOrderHold  Commented=on  SampleTime=0.0005
  PWM : Outport
  wires:
  Zero-Order Hold2/1 -> Saturation/1
  Constant1/1 -> Switch/3
  Constant/1 -> Switch/1
  Subtract2/1 -> Switch/2
  Repeating Sequence/1 -> Subtract2/2
  Saturation/1 -> Subtract2/1
  D/1 -> PWM Generator (DC-DC)/1
  PWM Generator (DC-DC)/1 -> PWM/1

== system rectifire_single_inverter_pv1/PV/T ==
  Demux : Demux  Tag=STV Demux  Outputs=1
      settings: DisplayOption=none
  FromWs : FromWorkspace  Tag=STV FromWs  VariableName=tuvar  ZeroCross=off
      SigBuilderData=|
      | dataSet.timeRange = [0 2]
      | dataSet.name = 'Group 1'
      | sbobj.Groups.Name = 'Group 1'
      | sbobj.Groups.Signals.Name = 'Signal 2'
      | sbobj.Groups.Signals.XData = [0 0.0805 0.16 2]
      | sbobj.Groups.Signals.YData = [25 20.1 25.01 25.01]
      | sbobj.Groups.TimeRange = [0 2]
  Signal 2 : Outport  Tag=STV Outport
  wires:
  FromWs/1 -> Demux/1
  Demux/1 -> Signal 2/1
